simulink model "exampleZufluss"  (Simulink 7.7)
settings: Solver=ode45  StartTime=0.0  StopTime=10.0  RelTol=1e-3
settings Model: Creator=hexren  LastModifiedBy=hexren

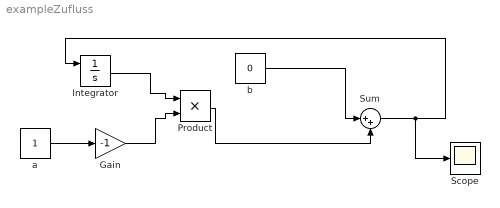
== system exampleZufluss ==
  Gain : Gain  Gain=-1
  Integrator : Integrator  InitialConditionSource=external
  Product : Product  RndMeth=Zero
  Scope : Scope
  Sum : Sum  Inputs=|++
  a : Constant
  b : Constant  Value=0
  wires:
  a/1 -> Gain/1
  Integrator/1 -> Product/1
  Gain/1 -> Product/2
  Product/1 -> Sum/2
  Sum/1 -> Integrator/1, Scope/1
  b/1 -> Sum/1
